simulink model "cessna_model"  (R2022b)
settings: Solver=VariableStepAuto  StartTime=0.0  StopTime=100  RelTol=1e-3
undefined symbols (not defined in the file or in its folder): DiscIntNeverNeededParam, Discrete, Earth, F, Light, MIL, Time, WGS84
libraries: aerolibtransform2 x3, sharedtransform x3, ctrlSharedLib x2, aerolibatmos2 x2, aerolibasang x1, aerolibpropulsion2 x1, slpidlib x1, uavalgslib x1, aerolibfltsims x1, dspstat3 x1, sensorgpslib x1, aerolibnav x1
settings Model: Creator=Muhammet  LastModifiedBy=Muhammet

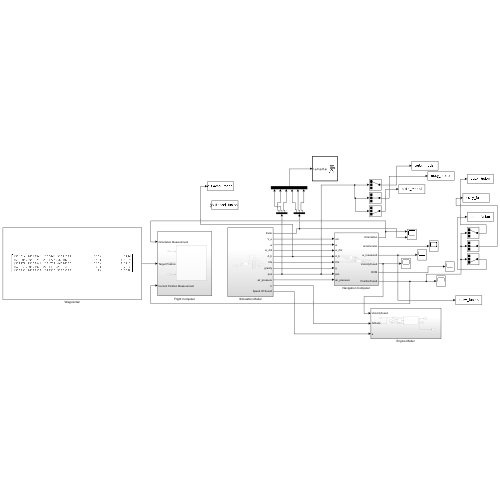
[thumbnail: Simulink's stored preview of the top-level diagram]
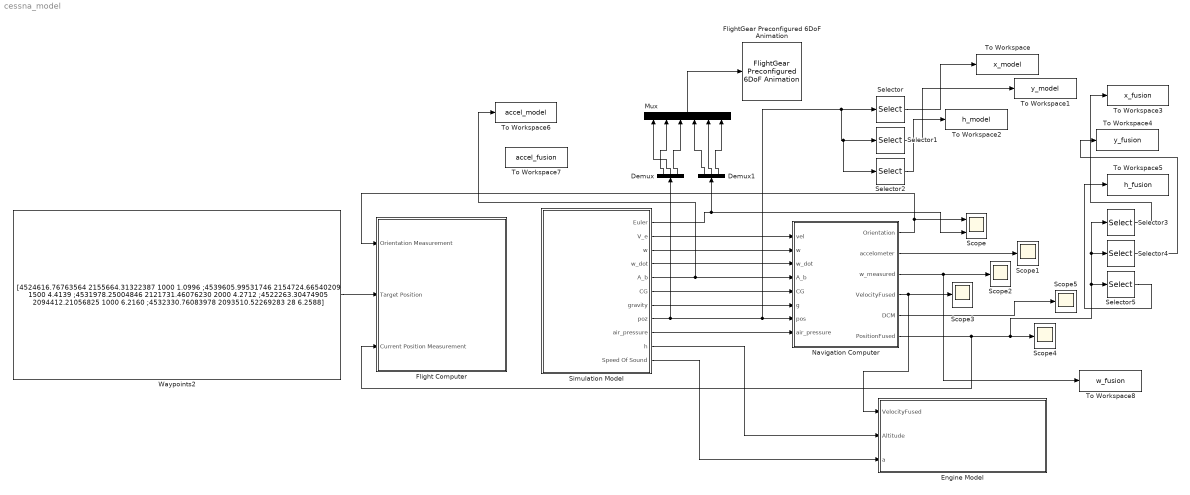
== system cessna_model ==
  Demux : Demux  Outputs=3
  Demux1 : Demux  Outputs=3
  "Engine Model " : Subsystem
  Flight Computer : Subsystem
  FlightGear Preconfigured 6DoF Animation : aerolibfltsims/FlightGear Preconfigured 6DoF Animation  xFlightGearVersion=v2019.1  DestinationIpAddress=127.0.0.1  DestinationPort=5502  SampleTime=1/30  packetVersion=24
  Mux : Mux  Inputs=6
  Navigation Computer : Subsystem
  Scope : Scope  NumInputPorts=2
  Scope{1..5} (5 alike) : Scope
  Selector : Selector  InputPortWidth=3  IndexOptions=Index vector (dialog)  Indices=[1]  OutputSizes=1
  Selector1 : Selector  InputPortWidth=3  IndexOptions=Index vector (dialog)  Indices=[2]  OutputSizes=1
  Selector2 : Selector  InputPortWidth=3  IndexOptions=Index vector (dialog)  Indices=[3]  OutputSizes=1
  Selector3 : Selector  InputPortWidth=3  IndexOptions=Index vector (dialog)  Indices=[1]  OutputSizes=1
  Selector4 : Selector  InputPortWidth=3  IndexOptions=Index vector (dialog)  Indices=[2]  OutputSizes=1
  Selector5 : Selector  InputPortWidth=3  IndexOptions=Index vector (dialog)  Indices=[3]  OutputSizes=1
  Simulation Model : Subsystem
  To Workspace : ToWorkspace  VariableName=x_model  SaveFormat=Timeseries  SampleTime=-1
  To Workspace1 : ToWorkspace  VariableName=y_model  SaveFormat=Timeseries  SampleTime=-1
  To Workspace2 : ToWorkspace  VariableName=h_model  SaveFormat=Timeseries  SampleTime=-1
  To Workspace3 : ToWorkspace  VariableName=x_fusion  SaveFormat=Timeseries  SampleTime=-1
  To Workspace4 : ToWorkspace  VariableName=y_fusion  SaveFormat=Timeseries  SampleTime=-1
  To Workspace5 : ToWorkspace  VariableName=h_fusion  SaveFormat=Timeseries  SampleTime=-1
  To Workspace6 : ToWorkspace  VariableName=accel_model  SaveFormat=Timeseries  SampleTime=-1
  To Workspace7 : ToWorkspace  VariableName=accel_fusion  SaveFormat=Timeseries  SampleTime=-1
  To Workspace8 : ToWorkspace  VariableName=w_fusion  SaveFormat=Timeseries  SampleTime=-1
  Waypoints2 : Constant  Value="[4524616.76763564 2155664.31322387 1000 1.0996 ;4539605.99531746\t2154724.66540209 1500  4.4139 ;4531978.25004846 2121731.46076230 2000  4.2712 ;4522263.30474905 2094412.21056825 1000  6.2160 ;4532330.76083978 2093510.52269283 28 6.2588]"
  wires:
  Navigation Computer/3(w_measured) -> To Workspace8/1, Scope2/1
  Demux1/2 -> Mux/5
  Simulation Model/1(Euler) -> Scope/2, Demux1/1
  Mux/1 -> FlightGear Preconfigured 6DoF Animation/1
  Simulation Model/6(CG) -> Navigation Computer/5(CG)
  Simulation Model/7(gravity) -> Navigation Computer/6(g)
  Navigation Computer/1(Orientation) -> Flight Computer/1(Orientation Measurement), Scope/1
  Demux1/1 -> Mux/4
  Demux/2 -> Mux/1
  Demux1/3 -> Mux/6
  Navigation Computer/2(accelometer) -> Scope1/1
  Simulation Model/9(air_pressure) -> Navigation Computer/8(air_pressure)
  Demux/1 -> Mux/2
  Simulation Model/8(poz) -> Demux/1, Selector2/1, Selector1/1, Selector/1, Navigation Computer/7(pos)
  Waypoints2/1 -> Flight Computer/2("Target Position ")
  Demux/3 -> Mux/3
  Navigation Computer/4(VelocityFused) -> "Engine Model "/1(VelocityFused), Scope3/1
  Navigation Computer/6(PositionFused) -> Flight Computer/3(Current Position Measurement), Selector5/1, Selector3/1, Selector4/1, Scope4/1
  Simulation Model/2(V_e) -> Navigation Computer/1(vel)
  Simulation Model/3(w) -> Navigation Computer/2(w)
  Simulation Model/4(w_dot) -> Navigation Computer/3(w_dot)
  Simulation Model/5(A_b) -> To Workspace6/1, Navigation Computer/4(A_b)
  Simulation Model/10(h) -> "Engine Model "/2(Altitude)
  Simulation Model/11(Speed Of Sound) -> "Engine Model "/3(a)
  Navigation Computer/5(DCM) -> Scope5/1
  Selector/1 -> To Workspace/1
  Selector1/1 -> To Workspace1/1
  Selector2/1 -> To Workspace2/1
  Selector3/1 -> To Workspace3/1
  Selector4/1 -> To Workspace4/1
  Selector5/1 -> To Workspace5/1

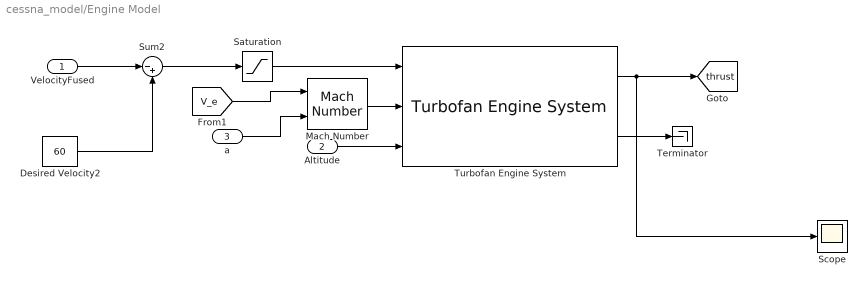
== system cessna_model/Engine Model  ==
  VelocityFused : Inport
  Altitude : Inport  Port=2
  a : Inport  Port=3
  Desired Velocity2 : Constant  Value=60
  Mach Number : aerolibasang/Mach Number
  Saturation : Saturate  UpperLimit=1  LowerLimit=0
  Scope : Scope
  Sum2 : Sum  Inputs=|-+
  Terminator : Terminator
  Turbofan Engine System : aerolibpropulsion2/Turbofan Engine System  units=Metric (MKS)  ic_source=Internal  IC=1  Fmax=400  tau=1  SFC=0.35  Nt=0.9
  tag scope: thrust=global
  wires:
  Turbofan Engine System/2 -> Terminator/1
  Turbofan Engine System/1 -> [thrust], Scope/1
  a/1 -> Mach Number/2
  Desired Velocity2/1 -> Sum2/2
  Mach Number/1 -> Turbofan Engine System/2
  Sum2/1 -> Saturation/1
  Altitude/1 -> Turbofan Engine System/3
  Saturation/1 -> Turbofan Engine System/1
  VelocityFused/1 -> Sum2/1
  [V_e] -> Mach Number/1

== system cessna_model/Flight Computer ==
  Orientation Measurement : Inport
  "Target Position " : Inport  Port=2
  Current Position Measurement : Inport  Port=3
  Flight Planner : Subsystem
  wires:
  Current Position Measurement/1 -> Flight Planner/1(currentpose)
  Orientation Measurement/1 -> Flight Planner/2(Orientation)
  "Target Position "/1 -> Flight Planner/3(In3)

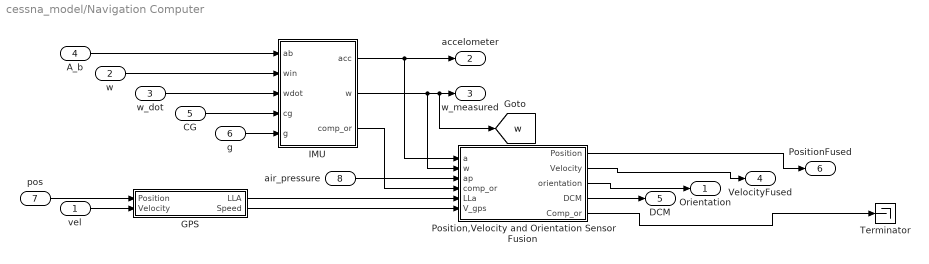
== system cessna_model/Navigation Computer ==
  vel : Inport
  w : Inport  Port=2
  w_dot : Inport  Port=3
  A_b : Inport  Port=4
  CG : Inport  Port=5
  g : Inport  Port=6
  pos : Inport  Port=7
  air_pressure : Inport  Port=8
  " Position,Velocity and Orientation Sensor Fusion" : Subsystem
  GPS : Subsystem
  IMU : Subsystem
  Terminator : Terminator
  Orientation : Outport
  accelometer : Outport  Port=2
  w_measured : Outport  Port=3
  VelocityFused : Outport  Port=4
  DCM : Outport  Port=5
  PositionFused : Outport  Port=6
  tag scope: w=global
  wires:
  " Position,Velocity and Orientation Sensor Fusion"/2(Velocity) -> VelocityFused/1
  " Position,Velocity and Orientation Sensor Fusion"/1(Position) -> PositionFused/1
  pos/1 -> GPS/1(Position)
  vel/1 -> GPS/2(Velocity)
  IMU/1(acc) -> " Position,Velocity and Orientation Sensor Fusion"/1(a), accelometer/1
  A_b/1 -> IMU/1(ab)
  w/1 -> IMU/2(win)
  w_dot/1 -> IMU/3(wdot)
  CG/1 -> IMU/4(cg)
  g/1 -> IMU/5(g)
  IMU/2(w) -> " Position,Velocity and Orientation Sensor Fusion"/2(w), [w], w_measured/1
  GPS/2(Speed) -> " Position,Velocity and Orientation Sensor Fusion"/6(V_gps)
  GPS/1(LLA) -> " Position,Velocity and Orientation Sensor Fusion"/5(LLa)
  air_pressure/1 -> " Position,Velocity and Orientation Sensor Fusion"/3(ap)
  " Position,Velocity and Orientation Sensor Fusion"/3(orientation) -> Orientation/1
  " Position,Velocity and Orientation Sensor Fusion"/4(DCM) -> DCM/1
  IMU/3(comp_or) -> " Position,Velocity and Orientation Sensor Fusion"/4(comp_or)
  " Position,Velocity and Orientation Sensor Fusion"/5(Comp_or) -> Terminator/1

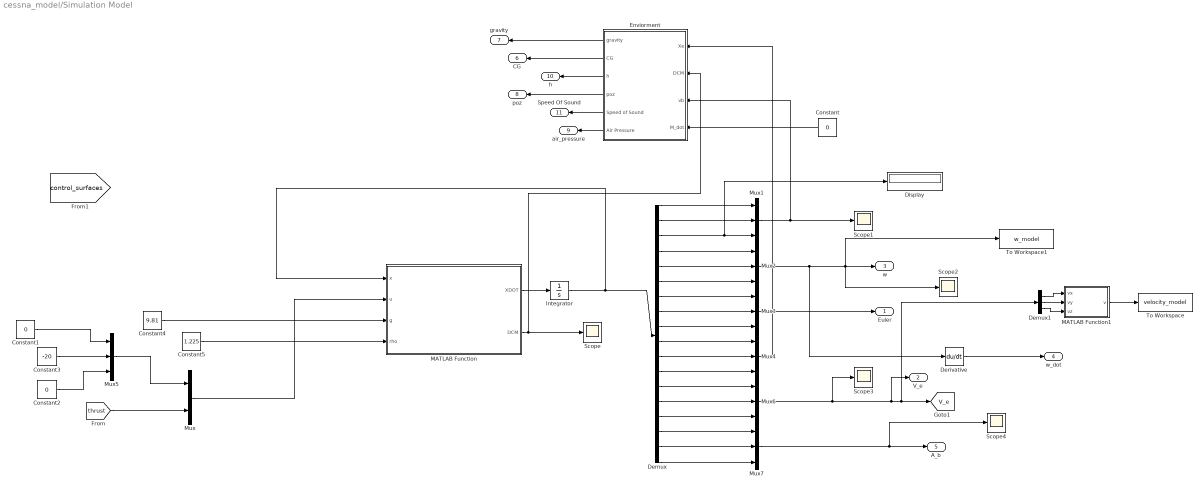
== system cessna_model/Simulation Model ==
  Constant : Constant  Value=0
  Constant1 : Constant  Value=0
  Constant2 : Constant  Value=0
  Constant3 : Constant  Value=-20
  Constant4 : Constant  Value=9.81
  Constant5 : Constant  Value=1.225
  Demux : Demux  Outputs=18
  Demux1 : Demux  Outputs=3
  Derivative : Derivative
  Display : Display
  Enviorment : Subsystem
  Integrator : Integrator  InitialCondition=[0;0.00000000000000000000000000001;0;0;0;0;0;0;1.09956;4521677.03993865; 2147705.52622961;-90;0;0;0;0;0;0;]
  MATLAB Function : MATLAB Function  TreatAsAtomicUnit=on
  MATLAB Function1 : MATLAB Function  TreatAsAtomicUnit=on
  Mux : Mux  Inputs=2
  Mux{1..7} (7 alike) : Mux  Inputs=3
  Scope{,1..4} (5 alike) : Scope
  To Workspace : ToWorkspace  VariableName=velocity_model  SaveFormat=Timeseries  SampleTime=-1
  To Workspace1 : ToWorkspace  VariableName=w_model  SaveFormat=Timeseries  SampleTime=-1
  Euler : Outport
  V_e : Outport  Port=2
  w : Outport  Port=3
  w_dot : Outport  Port=4
  A_b : Outport  Port=5
  CG : Outport  Port=6
  gravity : Outport  Port=7
  poz : Outport  Port=8
  air_pressure : Outport  Port=9
  h : Outport  Port=10
  Speed Of Sound : Outport  Port=11
  tag scope: V_e=global
  wires:
  Enviorment/1(gravity) -> gravity/1
  Enviorment/2(CG) -> CG/1
  Enviorment/3(h) -> h/1
  Enviorment/4(poz) -> poz/1
  Enviorment/5(Speed of Sound) -> Speed Of Sound/1
  Enviorment/6(Air Pressure) -> air_pressure/1
  Demux/14 -> Mux6/2
  Demux/13 -> Mux6/1
  Demux/6 -> Mux2/3
  Demux/18 -> Mux7/3
  Demux/10 -> Mux4/1
  Demux/3 -> Display/1, Mux1/3
  Demux/8 -> Mux3/2
  Demux/11 -> Mux4/2
  Demux/1 -> Mux1/1
  Demux/9 -> Mux3/3
  Demux/5 -> Mux2/2
  Demux/16 -> Mux7/1
  Demux/2 -> Mux1/2
  Demux/4 -> Mux2/1
  Demux/17 -> Mux7/2
  MATLAB Function/1(XDOT) -> Integrator/1
  MATLAB Function/2(DCM) -> Scope/1, Enviorment/2(DCM)
  Demux/15 -> Mux6/3
  Integrator/1 -> MATLAB Function/1(x), Demux/1
  Demux/7 -> Mux3/1
  Mux1/1 -> Enviorment/3(vb), Scope1/1
  Constant/1 -> Enviorment/4(M_dot)
  Mux2/1 -> Derivative/1, To Workspace1/1, Scope2/1, w/1
  Mux3/1 -> Euler/1
  Derivative/1 -> w_dot/1
  Mux7/1 -> Scope4/1, A_b/1
  Mux4/1 -> Enviorment/1(Xe)
  Mux6/1 -> Scope3/1, Demux1/1, [V_e], V_e/1
  Mux/1 -> MATLAB Function/2(u)
  Constant4/1 -> MATLAB Function/3(g)
  Constant5/1 -> MATLAB Function/4(rho)
  [thrust] -> Mux/2
  Demux/12 -> Mux4/3
  Mux5/1 -> Mux/1
  Constant2/1 -> Mux5/3
  Constant1/1 -> Mux5/1
  Constant3/1 -> Mux5/2
  Demux1/1 -> MATLAB Function1/1(vx)
  Demux1/2 -> MATLAB Function1/2(vy)
  Demux1/3 -> MATLAB Function1/3(vz)
  MATLAB Function1/1(v) -> To Workspace/1

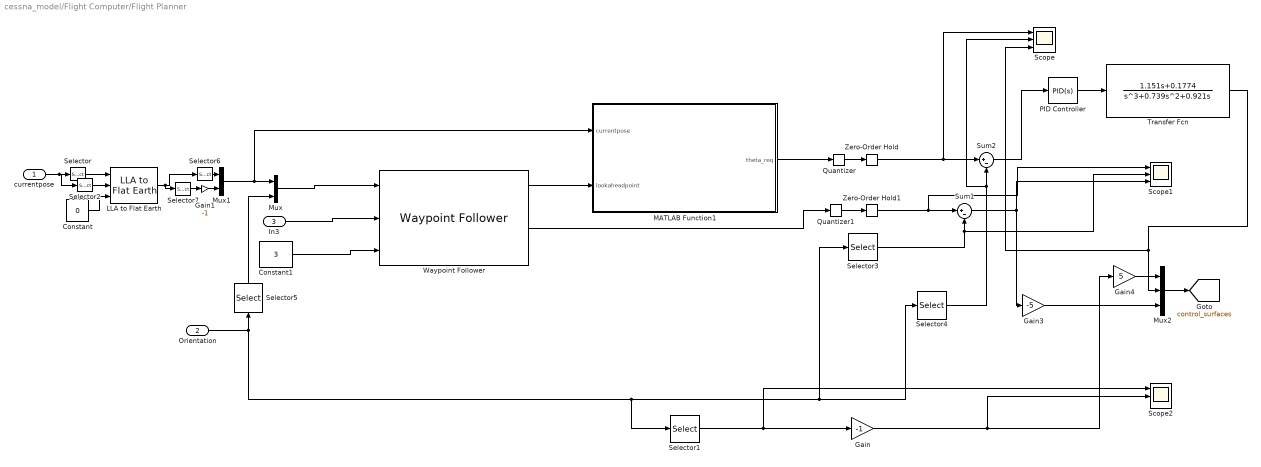
== system cessna_model/Flight Computer/Flight Planner ==
  currentpose : Inport
  Orientation : Inport  Port=2
  In3 : Inport  Port=3
  Constant : Constant  Value=0
  Constant1 : Constant  Value=3
  Gain : Gain  Gain=-1
  Gain1 : Gain  Gain=-1
  Gain3 : Gain  Gain=-5
  Gain4 : Gain  Gain=5
  LLA to Flat Earth : aerolibtransform2/LLA to Flat Earth  units=Metric (MKS)  ptype=Earth (WGS84)  F=1/298.257223563  R=6378137  refPosPort=off  LL0=[0 10]  psi=0
  MATLAB Function1 : MATLAB Function  TreatAsAtomicUnit=on
  Mux : Mux  Inputs=2
  Mux1 : Mux  Inputs=2
  Mux2 : Mux  Inputs=3
  PID Controller : slpidlib/PID Controller  Controller=PID  Form=Parallel  TimeDomain=Continuous-time  UseExternalTs=off  SampleTime=-1  IntegratorMethod=Forward Euler  FilterMethod=Forward Euler  ControllerParametersSource=internal  P=-0.543901899297658  I=-0.18196840813551  UseKiTs=off  D=0.286526504935986  N=0.562046268191802  UseFilter=on  TunerSelectOption=Transfer Function Based (PID Tuner App)  InitialConditionSource=internal  InitialConditionForIntegrator=0  InitialConditionForFilter=0  DifferentiatorICPrevScaledInput=0  ExternalReset=none  TrackingMode=off  Kt=1  LimitOutput=off  SatLimitsSource=internal  UpperSaturationLimit=inf  LowerSaturationLimit=-inf  LinearizeAsGain=on  AntiWindupMode=none  Kb=1  LimitIntegrator=off  UpperIntegratorSaturationLimit=inf  LowerIntegratorSaturationLimit=-inf  POutMin=[]  POutMax=[]  IOutMin=[]  IOutMax=[]  DOutMin=[]  DOutMax=[]  NOutMin=[]  NOutMax=[]  SumOutMin=[]  SumOutMax=[]  SaturationOutMin=[]  SaturationOutMax=[]  PParamMin=[]  PParamMax=[]  IParamMin=[]  IParamMax=[]  DParamMin=[]  DParamMax=[]  NParamMin=[]  NParamMax=[]  KbParamMin=[]  KbParamMax=[]  KtParamMin=[]  KtParamMax=[]  KbOutMin=[]  KbOutMax=[]  KtOutMin=[]  KtOutMax=[]  IntegratorOutMin=[]  IntegratorOutMax=[]  FilterOutMin=[]  FilterOutMax=[]  SumI1OutMin=[]  SumI1OutMax=[]  SumI2OutMin=[]  SumI2OutMax=[]  SumI3OutMin=[]  SumI3OutMax=[]  SumI4OutMin=[]  SumI4OutMax=[]  SumDOutMin=[]  SumDOutMax=[]  DifferentiatorOutMin=[]  DifferentiatorOutMax=[]  FilterDiffOutCoefMin=[]  FilterDiffOutCoefMax=[]  ReciprocalOutMin=[]  ReciprocalOutMax=[]  SumDenOutMin=[]  SumDenOutMax=[]  SumNumOutMin=[]  SumNumOutMax=[]  DivideOutMin=[]  DivideOutMax=[]  UdiffTsProdOutMin=[]  UdiffTsProdOutMax=[]  NTsProdOutMin=[]  NTsProdOutMax=[]  UintegralTsProdOutMin=[]  UintegralTsProdOutMax=[]  UngainTsProdOutMin=[]  UngainTsProdOutMax=[]  ClampingZeroOutDataTypeStr=Inherit: Inherit via back propagation  ClampingZeroOutMin=[]  ClampingZeroOutMax=[]  FilterDenConstantOutDataTypeStr=Inherit: Inherit via back propagation  FilterDenConstantOutMin=[]  FilterDenConstantOutMax=[]  PCopyOutDataTypeStr=Inherit: Inherit via back propagation  PCopyOutMin=[]  PCopyOutMax=[]  NCopyOutDataTypeStr=Inherit: Inherit via back propagation  NCopyOutMin=[]  NCopyOutMax=[]  IntegratorContinuousStateAttributes=''  IntegratorStateMustResolveToSignalObject=off  IntegratorRTWStateStorageClass=Auto  FilterContinuousStateAttributes=''  FilterStateMustResolveToSignalObject=off  FilterRTWStateStorageClass=Auto  ParallelPVariant=InternalParameters  IdealPVariant=Disabled  IVariant=InternalParameters  DVariant=InternalParameters  IntegratorVariant=Continuous  SatVariant=Disabled  AWVariant=Passthrough  PCopyVariant=Disabled  TRVariant=Disabled  FdbkBlocksVariant=Forward  IdealPFdbkVariant=Disabled  SatFdbkVariant=Disabled  DerivativeFilterVariant=ContFilter  NVariant=InternalParameters  NCopyVariant=Disabled  FilterICVariant=InternalICsFilter  IntegratorICVariant=InternalICs  ExternalResetVariant=Disabled  TRSumVariant=Passthrough  SumFdbkVariant=Disabled  SumVariant=Sum_PID  TsampFilterVariant=InternalTs  TsampNgainVariant=Passthrough  TsampIntegralVariant=Passthrough  ExternalSaturationOutDataTypeStr=Inherit: Same as second input
  Quantizer : Quantizer  QuantizationInterval=0.01
  Quantizer1 : Quantizer  QuantizationInterval=0.01
  Scope : Scope  NumInputPorts=3
  Scope1 : Scope  NumInputPorts=3
  Scope2 : Scope  NumInputPorts=3
  Selector : Selector  InputPortWidth=3  IndexOptions=Index vector (dialog)  Indices=[1 2]  OutputSizes=1
  Selector1 : Selector  InputPortWidth=3  IndexOptions=Index vector (dialog)  Indices=[1]  OutputSizes=1
  Selector{2..3,5,7} (4 alike) : Selector  InputPortWidth=3  IndexOptions=Index vector (dialog)  Indices=[3]  OutputSizes=1
  Selector4 : Selector  InputPortWidth=3  IndexOptions=Index vector (dialog)  Indices=[2]  OutputSizes=1
  Selector6 : Selector  InputPortWidth=3  IndexOptions=Index vector (dialog)  Indices=[1 2]  OutputSizes=1
  Sum1 : Sum  Inputs=|+-
  Sum2 : Sum  Inputs=|+-
  Transfer Fcn : TransferFcn  Numerator=[1.151 0.1774]  Denominator=[1 0.739 0.921 0]
  Waypoint Follower : uavalgslib/Waypoint Follower  UAVType=fixed-wing  StartFrom=first  TransitionRadiusSource=internal  TransitionRadius=10  MinLookaheadDistance=0.5  YawInput=on  ShowCrossTrackErrorOutput=off  ShowStatusOutput=off  SimulateUsing=Interpreted execution
  Zero-Order Hold : ZeroOrderHold  SampleTime=-1
  Zero-Order Hold1 : ZeroOrderHold  SampleTime=-1
  tag scope: control_surfaces=global
  wires:
  In3/1 -> Waypoint Follower/2
  Selector5/1 -> Mux/2
  Mux/1 -> Waypoint Follower/1
  Constant1/1 -> Waypoint Follower/3
  currentpose/1 -> Selector/1, Selector2/1
  Selector/1 -> LLA to Flat Earth/1
  Selector2/1 -> LLA to Flat Earth/2
  Constant/1 -> LLA to Flat Earth/3
  Mux1/1 -> MATLAB Function1/1(currentpose), Mux/1
  LLA to Flat Earth/1 -> Selector6/1, Selector7/1
  Selector6/1 -> Mux1/1
  Selector7/1 -> Gain1/1
  Gain1/1 -> Mux1/2
  Quantizer/1 -> Zero-Order Hold/1
  Waypoint Follower/3 -> Quantizer1/1
  Quantizer1/1 -> Zero-Order Hold1/1
  Zero-Order Hold/1 -> Scope/1, Sum2/1
  Selector3/1 -> Scope1/2, Sum1/2
  Selector1/1 -> Scope2/1, Gain/1
  MATLAB Function1/1(theta_req) -> Quantizer/1
  Orientation/1 -> Selector5/1, Selector1/1, Selector4/1, Selector3/1
  Zero-Order Hold1/1 -> Scope1/1, Sum1/1
  Selector4/1 -> Scope/2, Sum2/2
  Waypoint Follower/1 -> MATLAB Function1/2(lookaheadpoint)
  Mux2/1 -> [control_surfaces]
  Gain/1 -> Scope2/2, Gain4/1
  Transfer Fcn/1 -> Scope/3, Mux2/2
  Gain3/1 -> Mux2/3
  Gain4/1 -> Mux2/1
  Sum1/1 -> Gain3/1, Scope1/3
  PID Controller/1 -> Transfer Fcn/1
  Sum2/1 -> PID Controller/1

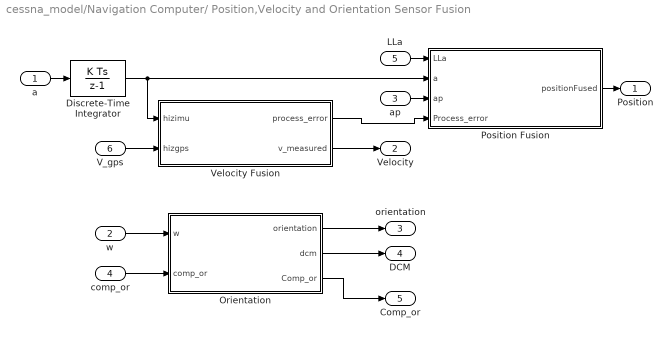
== system cessna_model/Navigation Computer/ Position,Velocity and Orientation Sensor Fusion ==
  a : Inport
  w : Inport  Port=2
  ap : Inport  Port=3
  comp_or : Inport  Port=4
  LLa : Inport  Port=5
  V_gps : Inport  Port=6
  Discrete-Time Integrator : DiscreteIntegrator  SampleTime=-1  ICPrevOutput=DiscIntNeverNeededParam  ICPrevScaledInput=DiscIntNeverNeededParam
  Orientation : Subsystem
  Position Fusion : Subsystem
  Velocity Fusion : Subsystem
  Position : Outport
  Velocity : Outport  Port=2
  orientation : Outport  Port=3
  DCM : Outport  Port=4
  Comp_or : Outport  Port=5
  wires:
  a/1 -> Discrete-Time Integrator/1
  Discrete-Time Integrator/1 -> Velocity Fusion/1(hizimu), Position Fusion/2(a)
  LLa/1 -> Position Fusion/1(LLa)
  ap/1 -> Position Fusion/3(ap)
  Position Fusion/1(positionFused) -> Position/1
  Velocity Fusion/1(process_error) -> Position Fusion/4(Process_error)
  Velocity Fusion/2(v_measured) -> Velocity/1
  V_gps/1 -> Velocity Fusion/2(hizgps)
  w/1 -> Orientation/1(w)
  Orientation/1(orientation) -> orientation/1
  Orientation/2(dcm) -> DCM/1
  comp_or/1 -> Orientation/2(comp_or)
  Orientation/3(Comp_or) -> Comp_or/1

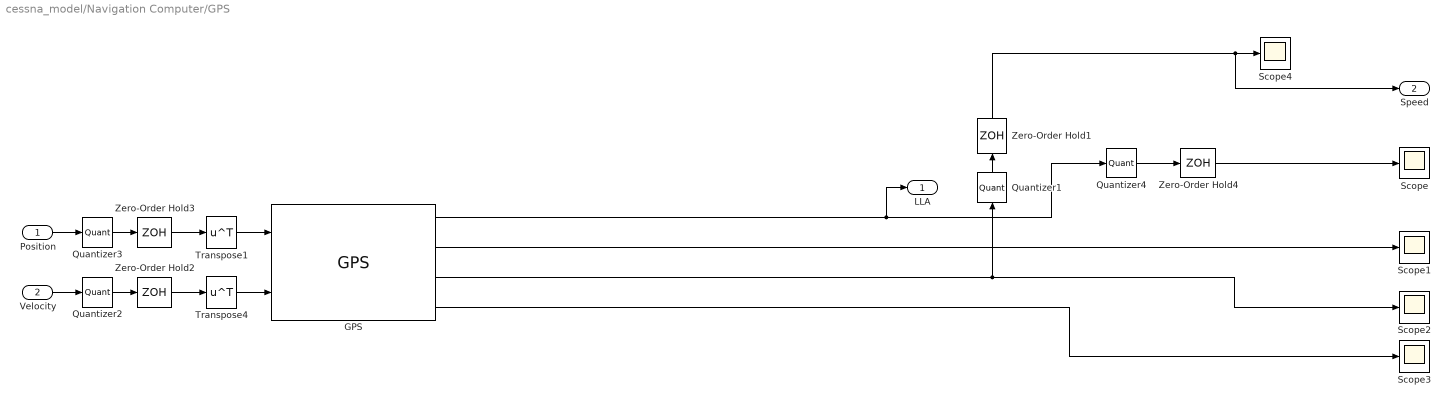
== system cessna_model/Navigation Computer/GPS ==
  Position : Inport
  Velocity : Inport  Port=2
  GPS : sensorgpslib/GPS  DispRefFrame=NED  PositionInputFormat=Geodetic  ReferenceLocation=[ 0, 0, 0 ]  HorizontalPositionAccuracy=0  VerticalPositionAccuracy=0  VelocityAccuracy=0  DecayFactor=0.999  SeedDouble=0  SimulateUsing=Interpreted execution
  Quantizer{1..4} (4 alike) : Quantizer  QuantizationInterval=0.01
  Scope{,1..4} (5 alike) : Scope
  Transpose1 : Math  Operator=transpose
  Transpose4 : Math  Operator=transpose
  Zero-Order Hold{1..4} (4 alike) : ZeroOrderHold  SampleTime=-1
  LLA : Outport
  Speed : Outport  Port=2
  wires:
  Velocity/1 -> Quantizer2/1
  GPS/2 -> Scope1/1
  Position/1 -> Quantizer3/1
  GPS/3 -> Scope2/1, Quantizer1/1
  GPS/4 -> Scope3/1
  GPS/1 -> LLA/1, Quantizer4/1
  Transpose1/1 -> GPS/1
  Transpose4/1 -> GPS/2
  Quantizer1/1 -> Zero-Order Hold1/1
  Zero-Order Hold1/1 -> Speed/1, Scope4/1
  Quantizer3/1 -> Zero-Order Hold3/1
  Zero-Order Hold3/1 -> Transpose1/1
  Quantizer2/1 -> Zero-Order Hold2/1
  Zero-Order Hold2/1 -> Transpose4/1
  Quantizer4/1 -> Zero-Order Hold4/1
  Zero-Order Hold4/1 -> Scope/1

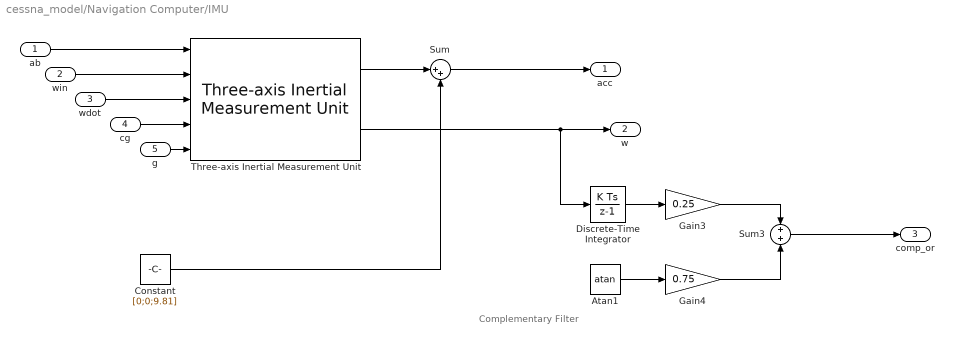
== system cessna_model/Navigation Computer/IMU ==
  note: Complementary Filter
  ab : Inport
  win : Inport  Port=2
  wdot : Inport  Port=3
  cg : Inport  Port=4
  g : Inport  Port=5
  Atan1 : Trigonometry  Operator=atan
  Constant : Constant  Value=[0;0;9.81]
  Discrete-Time Integrator : DiscreteIntegrator  InitialCondition=|  SampleTime=-1  ICPrevOutput=DiscIntNeverNeededParam  ICPrevScaledInput=DiscIntNeverNeededParam
      | [0 0 1.0996
      | ]
  Gain3 : Gain  Gain=0.25
  Gain4 : Gain  Gain=0.75
  Sum : Sum  Inputs=|++
  Sum3 : Sum
  Three-axis Inertial Measurement Unit : aerolibnav/Three-axis Inertial Measurement Unit  units=Metric (MKS)  imu=[0 0 0]  i_Ts=0.01  dtype_a=on  w_a=190  z_a=0.707  a_sf_cc=[1 0 0; 0 1 0; 0 0 1]  a_bias=[0 0 0]  a_sat="[-inf  -inf  -inf  inf inf inf]"  dtype_g=on  w_g=190  z_g=0.707  g_sf_cc=[1 0 0; 0 1 0; 0 0 1]  g_bias=[0 0 0]  g_sens=[0 0 0]  g_sat="[-inf  -inf  -inf  inf inf inf]"  i_rand=off  i_seeds=[23093 23094 23095 23096 23097 23098]  i_pow=[0.0001 0.0001 0.0001 0.0001 0.0001 0.0001]
  acc : Outport
  w : Outport  Port=2
  comp_or : Outport  Port=3
  wires:
  win/1 -> Three-axis Inertial Measurement Unit/2
  wdot/1 -> Three-axis Inertial Measurement Unit/3
  cg/1 -> Three-axis Inertial Measurement Unit/4
  g/1 -> Three-axis Inertial Measurement Unit/5
  Discrete-Time Integrator/1 -> Gain3/1
  Gain3/1 -> Sum3/1
  Gain4/1 -> Sum3/2
  Atan1/1 -> Gain4/1
  Sum3/1 -> comp_or/1
  Three-axis Inertial Measurement Unit/2 -> w/1, Discrete-Time Integrator/1
  ab/1 -> Three-axis Inertial Measurement Unit/1
  Three-axis Inertial Measurement Unit/1 -> Sum/1
  Constant/1 -> Sum/2
  Sum/1 -> acc/1

== system cessna_model/Simulation Model/Enviorment ==
  Xe : Inport
  DCM : Inport  Port=2
  vb : Inport  Port=3
  M_dot : Inport  Port=4
  Atmosphere Model : Subsystem
  Gravity Model : Subsystem
  gravity : Outport
  CG : Outport  Port=2
  h : Outport  Port=3
  poz : Outport  Port=4
  Speed of Sound : Outport  Port=5
  Air Pressure : Outport  Port=6
  wires:
  Gravity Model/4(h) -> h/1, Atmosphere Model/1(Altitude)
  vb/1 -> Atmosphere Model/3(vb)
  Gravity Model/3(poz) -> poz/1
  M_dot/1 -> Gravity Model/2(M_dot)
  Atmosphere Model/3(Air Pressure) -> Air Pressure/1
  Atmosphere Model/1(Temperature) -> ?
  Xe/1 -> Gravity Model/1(Xe)
  DCM/1 -> Atmosphere Model/2(DCM)
  Atmosphere Model/2(Speed of Sound) -> Speed of Sound/1
  Gravity Model/1(gravity) -> gravity/1
  Gravity Model/2(CG) -> CG/1

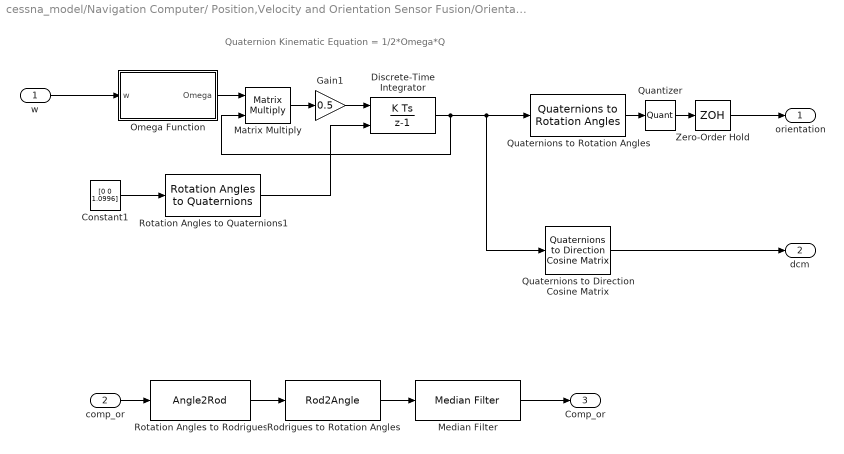
== system cessna_model/Navigation Computer/ Position,Velocity and Orientation Sensor Fusion/Orientation ==
  note: Quaternion Kinematic Equation = 1/2*Omega*Q
  w : Inport
  comp_or : Inport  Port=2
  Constant1 : Constant  Value=[0 0 1.0996]
  Discrete-Time Integrator : DiscreteIntegrator  InitialConditionSource=external  SampleTime=0.01  ICPrevOutput=DiscIntNeverNeededParam  ICPrevScaledInput=DiscIntNeverNeededParam
  Gain1 : Gain  Gain=0.5
  Matrix Multiply : Product  Multiplication=Matrix(*)
  Median Filter : dspstat3/Median Filter  WindowLength=5  SimulateUsing=Interpreted execution
      settings: LibrarySourceBlock=|
      | dspfdesign/Median
      | Filter
  Omega Function : MATLAB Function  TreatAsAtomicUnit=on
  Quantizer : Quantizer  QuantizationInterval=0.01  LinearizeAsGain=off
  Quaternions to Direction Cosine Matrix : sharedtransform/Quaternions to  Direction Cosine Matrix  aMode=aMode
  Quaternions to Rotation Angles : sharedtransform/Quaternions to Rotation Angles  rotationOrder=XYZ  aMode=aMode
  Rodrigues to Rotation Angles : Rod2Angle  rotationOrder=XYZ
      settings: AttributesFormatString=Rotation Order: %<rotationOrder>
  Rotation Angles to Quaternions1 : sharedtransform/Rotation Angles to Quaternions  rotationOrder=XYZ  aMode=aMode
  Rotation Angles to Rodrigues : Angle2Rod  rotationOrder=XYZ
      settings: AttributesFormatString=Rotation Order: %<rotationOrder>
  Zero-Order Hold : ZeroOrderHold  SampleTime=-1
  orientation : Outport
  dcm : Outport  Port=2
  Comp_or : Outport  Port=3
  wires:
  Quaternions to Direction Cosine Matrix/1 -> dcm/1
  Constant1/1 -> Rotation Angles to Quaternions1/1
  Rotation Angles to Quaternions1/1 -> Discrete-Time Integrator/2
  w/1 -> Omega Function/1(w)
  Gain1/1 -> Discrete-Time Integrator/1
  Discrete-Time Integrator/1 -> Matrix Multiply/2, Quaternions to Rotation Angles/1, Quaternions to Direction Cosine Matrix/1
  Matrix Multiply/1 -> Gain1/1
  Omega Function/1(Omega) -> Matrix Multiply/1
  comp_or/1 -> Rotation Angles to Rodrigues/1
  Rotation Angles to Rodrigues/1 -> Rodrigues to Rotation Angles/1
  Rodrigues to Rotation Angles/1 -> Median Filter/1
  Quaternions to Rotation Angles/1 -> Quantizer/1
  Median Filter/1 -> Comp_or/1
  Quantizer/1 -> Zero-Order Hold/1
  Zero-Order Hold/1 -> orientation/1

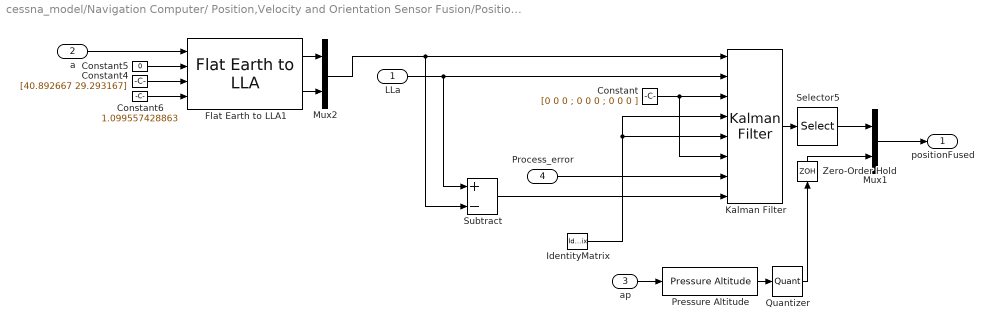
== system cessna_model/Navigation Computer/ Position,Velocity and Orientation Sensor Fusion/Position Fusion ==
  LLa : Inport
  a : Inport  Port=2
  ap : Inport  Port=3
  Process_error : Inport  Port=4
  Constant : Constant  Value=[0 0 0 ; 0 0 0 ; 0 0 0 ]  SampleTime=0.01
  Constant4 : Constant  Value=[40.892667 29.293167]
  Constant5 : Constant  Value=0
  Constant6 : Constant  Value=1.099557428863
  Flat Earth to LLA1 : aerolibtransform2/Flat Earth to LLA  units=Metric (MKS)  ptype=Earth (WGS84)  F=1/298.257223563  R=6378137  refPosPort=on  LL0=[0 10]  psi=0
  IdentityMatrix : IdentityMatrix  OutputDimensions=3  SampleTime=0.01
  Kalman Filter : ctrlSharedLib/Kalman Filter  TimeDomain=Discrete-Time  UseCurrentEstimator=on  ModelSource=Input port  ModelSourceVariable=ss(0.95,1,1,0,1)  A=0.95  B=1  C=1  D=0  NumberOfStates=3  NumberOfInputs=3  NumberOfOutputs=3  InitialEstimateSource=Dialog  X0=0  P0=10  UseK=off  UseGH=off  NumberOfProcessNoiseInputs=1  G=1  TimeInvariantG=on  H=0  TimeInvariantH=on  Q=0.05  TimeInvariantQ=off  R=1  TimeInvariantR=off  N=0  TimeInvariantN=on  AddInputPort=on  AddEnablePort=off  OutputEstimatedY=off  OutputP=off  Ts=0.01
  Mux1 : Mux  Inputs=2
  Mux2 : Mux  Inputs=2
  Pressure Altitude : aerolibatmos2/Pressure Altitude  units=Metric (MKS)  action=Warning
  Quantizer : Quantizer  QuantizationInterval=0.01
  Selector5 : Selector  InputPortWidth=3  IndexOptions=Index vector (dialog)  Indices=[1 2]  OutputSizes=1
  Subtract : Sum  Inputs=+-
  Zero-Order Hold : ZeroOrderHold  SampleTime=-1
  positionFused : Outport
  wires:
  LLa/1 -> Subtract/1, Kalman Filter/2
  Subtract/1 -> Kalman Filter/8
  Mux1/1 -> positionFused/1
  Selector5/1 -> Mux1/1
  IdentityMatrix/1 -> Kalman Filter/5, Kalman Filter/4
  Kalman Filter/1 -> Selector5/1
  Process_error/1 -> Kalman Filter/7
  Constant/1 -> Kalman Filter/6, Kalman Filter/3
  Pressure Altitude/1 -> Quantizer/1
  ap/1 -> Pressure Altitude/1
  Quantizer/1 -> Zero-Order Hold/1
  Zero-Order Hold/1 -> Mux1/2
  Mux2/1 -> Subtract/2, Kalman Filter/1
  Constant5/1 -> Flat Earth to LLA1/2
  Flat Earth to LLA1/1 -> Mux2/1
  Constant6/1 -> Flat Earth to LLA1/4
  a/1 -> Flat Earth to LLA1/1
  Constant4/1 -> Flat Earth to LLA1/3
  Flat Earth to LLA1/2 -> Mux2/2

== system cessna_model/Navigation Computer/ Position,Velocity and Orientation Sensor Fusion/Velocity Fusion ==
  hizimu : Inport
  hizgps : Inport  Port=2
  Constant1 : Constant  Value=0
  Demux : Demux  Outputs=3
  IdentityMatrix1 : IdentityMatrix  OutputDimensions=1  SampleTime=0.01
  Kalman Filter1 : ctrlSharedLib/Kalman Filter  TimeDomain=Discrete-Time  UseCurrentEstimator=on  ModelSource=Input port  ModelSourceVariable=ss(0.95,1,1,0,1)  A=0.95  B=1  C=1  D=0  NumberOfStates=1  NumberOfInputs=1  NumberOfOutputs=1  InitialEstimateSource=Dialog  X0=0  P0=10  UseK=off  UseGH=off  NumberOfProcessNoiseInputs=1  G=1  TimeInvariantG=on  H=0  TimeInvariantH=on  Q=0.05  TimeInvariantQ=off  R=1  TimeInvariantR=on  N=0  TimeInvariantN=on  AddInputPort=on  AddEnablePort=off  OutputEstimatedY=off  OutputP=off  Ts=0.01
  MATLAB Function : MATLAB Function  TreatAsAtomicUnit=on
  Sum : Sum  Inputs=|+-
  To Workspace : ToWorkspace  VariableName=velocity_fusion  SaveFormat=Timeseries  SampleTime=-1
  process_error : Outport
  v_measured : Outport  Port=2
  wires:
  Demux/1 -> MATLAB Function/1(vx)
  Demux/2 -> MATLAB Function/2(vy)
  Constant1/1 -> Kalman Filter1/6, Kalman Filter1/3
  Demux/3 -> MATLAB Function/3(vz)
  hizimu/1 -> Demux/1
  IdentityMatrix1/1 -> Kalman Filter1/4, Kalman Filter1/5
  MATLAB Function/1(v) -> Kalman Filter1/2, Sum/2
  Sum/1 -> process_error/1, Kalman Filter1/7
  Kalman Filter1/1 -> To Workspace/1, v_measured/1
  hizgps/1 -> Kalman Filter1/1, Sum/1

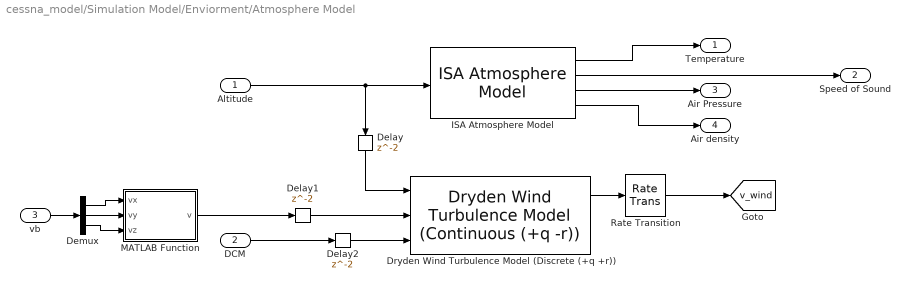
== system cessna_model/Simulation Model/Enviorment/Atmosphere Model ==
  Altitude : Inport
  DCM : Inport  Port=2
  vb : Inport  Port=3
  Delay : Delay
  Delay1 : Delay
  Delay2 : Delay
  Demux : Demux  Outputs=3
  Dryden Wind Turbulence Model (Discrete (+q +r)) : aerolibwind2/Dryden Wind Turbulence Model  (Continuous (+q -r))  units=Metric (MKS)  spec=MIL-F-8785C  model=Discrete Dryden (+q +r)  W20=0  Wdeg=0  TurbProb=10^-2 - Light  L_high=533.4  Wingspan=11  ts=0.1  Seed=[23341 23342 23343 23344]  T_on=on
      settings: LibrarySourceBlock=|
      | aerolibwind2/Dryden Wind Turbulence Model
      | (Discrete (+q +r))
  ISA Atmosphere Model : aerolibatmos2/ISA Atmosphere Model  custom=off  g=9.80665  gamma=1.4  R=287.0531  L=0.0065  h_trop=11000  h_strat=20000  rho0=1.225  P0=101325  T0=288.15  h0=0
  MATLAB Function : MATLAB Function  TreatAsAtomicUnit=on
  Rate Transition : RateTransition  OutPortSampleTime=0
  Temperature : Outport
  Speed of Sound : Outport  Port=2
  Air Pressure : Outport  Port=3
  Air density : Outport  Port=4
  tag scope: v_wind=global
  wires:
  ISA Atmosphere Model/2 -> Speed of Sound/1
  Altitude/1 -> Delay/1, ISA Atmosphere Model/1
  ISA Atmosphere Model/1 -> Temperature/1
  ISA Atmosphere Model/4 -> Air density/1
  ISA Atmosphere Model/3 -> Air Pressure/1
  DCM/1 -> Delay2/1
  Demux/1 -> MATLAB Function/1(vx)
  Demux/2 -> MATLAB Function/2(vy)
  Demux/3 -> MATLAB Function/3(vz)
  MATLAB Function/1(v) -> Delay1/1
  vb/1 -> Demux/1
  Delay/1 -> Dryden Wind Turbulence Model (Discrete (+q +r))/1
  Delay1/1 -> Dryden Wind Turbulence Model (Discrete (+q +r))/2
  Delay2/1 -> Dryden Wind Turbulence Model (Discrete (+q +r))/3
  Dryden Wind Turbulence Model (Discrete (+q +r))/1 -> Rate Transition/1
  Rate Transition/1 -> [v_wind]

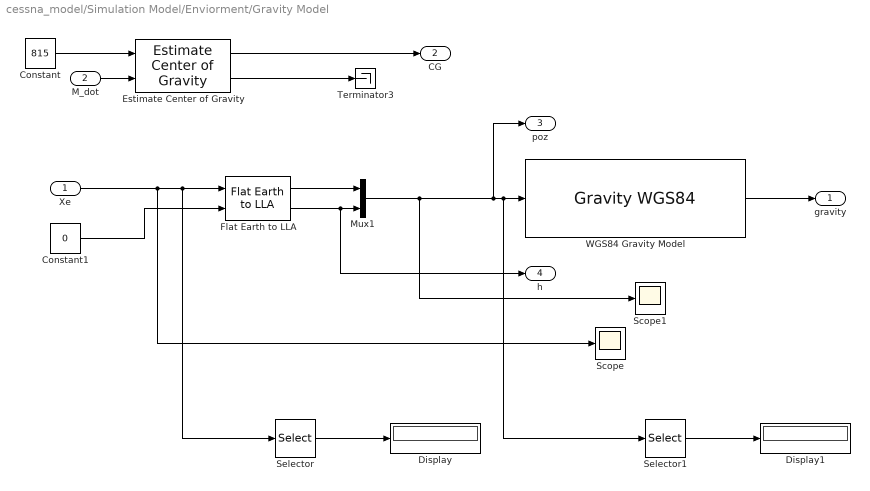
== system cessna_model/Simulation Model/Enviorment/Gravity Model ==
  Xe : Inport
  M_dot : Inport  Port=2
  Constant : Constant  Value=815
  Constant1 : Constant  Value=0
  Display : Display
  Display1 : Display
  Estimate Center of Gravity : aerolibbdyn/Estimate Center of Gravity  fmass=800 + 105  emass=800  fcg=[7 1.27 1.36]'  ecg=[7 1.27 1.36]'
  Flat Earth to LLA : aerolibtransform2/Flat Earth to LLA  units=Metric (MKS)  ptype=Earth (WGS84)  F=1/298.257223563  R=6378137  refPosPort=off  LL0=[0 10]  psi=0
  Mux1 : Mux  Inputs=2
  Scope : Scope
  Scope1 : Scope
  Selector : Selector  InputPortWidth=3  IndexOptions=Index vector (dialog)  Indices=[3]  OutputSizes=1
  Selector1 : Selector  InputPortWidth=3  IndexOptions=Index vector (dialog)  Indices=[3]  OutputSizes=1
  Terminator3 : Terminator
  "WGS84 Gravity Model  " : GravityWGS84
  gravity : Outport
  CG : Outport  Port=2
  poz : Outport  Port=3
  h : Outport  Port=4
  wires:
  Mux1/1 -> Selector1/1, "WGS84 Gravity Model  "/1, poz/1, Scope1/1
  M_dot/1 -> Estimate Center of Gravity/2
  Estimate Center of Gravity/2 -> Terminator3/1
  Constant/1 -> Estimate Center of Gravity/1
  Estimate Center of Gravity/1 -> CG/1
  "WGS84 Gravity Model  "/1 -> gravity/1
  Xe/1 -> Selector/1, Flat Earth to LLA/1, Scope/1
  Constant1/1 -> Flat Earth to LLA/2
  Flat Earth to LLA/1 -> Mux1/1
  Flat Earth to LLA/2 -> h/1, Mux1/2
  Selector/1 -> Display/1
  Selector1/1 -> Display1/1

== matlab function cessna_model/Simulation Model/MATLAB Function1 ==
  data: vx input; v output; vy input; vz input
function v = fcn(vx, vy, vz)
v = sqrt((vx^2)+(vy^2)+(vz^2));

== matlab function cessna_model/Navigation Computer/ Position,Velocity and Orientation Sensor Fusion/Velocity Fusion/MATLAB Function ==
  data: vx input; v output; vy input; vz input
function v = fcn(vx, vy, vz)
v = sqrt((vx^2)+(vy^2)+(vz^2));

== matlab function cessna_model/Simulation Model/MATLAB Function ==
  data: x input; u input; g input; rho input; XDOT output; DCM output
function [XDOT,DCM] = cessna_model_xdot(x,u,g,rho)

x1=x(1);    %u
x2=x(2);    %v
x3=x(3);    %w
x4=x(4);    %p
x5=x(5);    %q
x6=x(6);    %r
x7=x(7);    %phi
x8=x(8);    %theta
x9=x(9);    %psi
x10=x(10);  %x
x11=x(11);  %y
x12=x(12);  %z

u1=u(1);    % Aileron Input (Deflection)
u2=u(2);    % Elevator Input (Deflection)
u3=u(3);    % Rudder Input   (Deflection)
u4=u(4);    % Thrust In Newtons


m = 815 ; % Mass
Inertia = [1285.3154279 0 -161.5 ; 0 1824.9309767 0 ; -161.5 0 2666.893931];
S = 16; % Wing Area
Cbar = 1.45; % Mean Aerodynamic Chord
b = 11; % Winspan

Va = sqrt((x1^2)+(x2^2)+(x3^2)); % Airspeed

alphar = atan2(x3,x1);   %Angle of Attack
alpha=rad2deg(alphar);
betar = asin(x2/Va);     %Angle of Sideslip
beta =rad2deg(betar);
qbar = 0.5*rho*Va^2;    %Dynamic Pressure


C1 = [cos(x9) sin(x9) 0 ; -sin(x9) cos(x9) 0 ; 0 0 1];
C2 = [cos(x8) 0 -sin(x8);0 1 0 ; sin(x8) 0 cos(x8)];  % DCM
C3 = [1 0 0 ; 0 cos(x7) sin(x7); 0 -sin(x7) cos(x7)];
Cw_b = C1*C2*C3;
DCM = transpose(Cw_b);


u1max = 10*pi/180;
u1min =-10*pi/180;
u2max = 20*pi/180;    % Control Surface Limits
u2min =-20*pi/180;
u3max = 10*pi/180;
u3min =-10*pi/180;

if(u1>u1max)
    u1=u1max;
elseif(u1<u1min)        % Control Saturations
    u1=u1min;
end
if(u2>u2max)
    u2=u2max;
elseif(u2<u2min)
    u2=u2min;
end
if(u3>u3max)
    u3=u3max;
elseif(u3<u3min)
    u3=u3min;
end

Ct = 0.031;
CD = (0.031+0.13*alpha+0.06*u2);
CL = (5.143*alpha+0.43*u2+0.31+3.9*x5); % Aerodynamic Force And Moment Stability Coefficients
Clm = (0.178*u1+0.0147*u3-0.047*x4);
Cmm = (-0.89*alpha-12.4*x5-1.28*u2);
Cnm = (0.065*beta-0.099*x6-0.0657*u3);

CX = -CD*cos(alpha)+CL*sin(alpha);    
CY = (-0.31*beta+0.187*u3);        % Force Coefficients
CZ = -CD*sin(alpha)-CL*cos(alpha);

%Translational Accelerations On Body
Xab = (CX*qbar*S+Ct*u4)/m;
Yab = (CY*qbar*S)/m;
Zab = (CZ*qbar*S)/m;

x16to18dot=[Xab;Yab;Zab];

%Rotational Accelerations On Body
Lb = Clm*qbar*S*b;
Mb = Cmm*qbar*S*Cbar;
Nb = Cnm*qbar*S*b;
Load_Factor = Zab/g;

% Equations Of Motion
Udot = Xab + (x6*x2-x2*x5)*g*cos(x8);
Vdot = Yab + (x4*x3-x1*x6)*sin(x7)*cos(x8);
Wdot = Zab + (x5*x1-x4*x2)*cos(x7)*cos(x8);
x1to3dot = [Udot;Vdot;Wdot];

Pdot = Lb/1285.3154279 ;
Qdot = (Mb+(2666.893931-1285.3154279)*x4*x6)/1824.9309767;
Rdot = (Nb+(1285.3154279-1824.9309767)*x4*x5)/2666.893931;
x4to6dot=[Pdot;Qdot;Rdot];
Wbe = [x4;x5;x6];
% Euler Angles
x7to9dot=[1 sin(x7)*tan(x8) cos(x7)*tan(x8);0 cos(x7) -sin(x7);0 sin(x7)*cos(x8) cos(x7)*cos(x8)]*Wbe;
V_b = [x1;x2;x3];

% Position 
x10to12dot=DCM*V_b;

% Velocities on Earth Frame
x13to15dot=DCM*V_b;


XDOT=[x1to3dot;x4to6dot;x7to9dot;x10to12dot;x13to15dot;x16to18dot];

== matlab function cessna_model/Simulation Model/Enviorment/Atmosphere Model/MATLAB Function ==
  data: vx input; v output; vy input; vz input
function v = fcn(vx, vy, vz)
v = sqrt((vx^2)+(vy^2)+(vz^2));

== matlab function cessna_model/Navigation Computer/ Position,Velocity and Orientation Sensor Fusion/Orientation/Omega Function ==
  data: w input; Omega output
function Omega = fcn(w)
wx=w(1)
wy=w(2)
wz=w(3)

Omega = [0 -wx -wy -wz;
        wx 0 wz -wy;
        wy -wz 0 wx;
        wz wy -wx 0];

== matlab function cessna_model/Flight Computer/Flight Planner/MATLAB Function1 ==
  data: currentpose input; lookaheadpoint input; theta_req output
function theta_req = fcn(currentpose,lookaheadpoint)
x2=lookaheadpoint(1);
x1=currentpose(1);
y2=lookaheadpoint(2);
y1=currentpose(2);
z2=lookaheadpoint(3);
z1=currentpose(3);

dz = sqrt([x2-x1]^2+[y2-y1]^2);
h_opposite=z2-z1;

theta_req=tan(h_opposite/dz);
psi_req= sin((y2-y1)/dz);
